simulink model "PhyMod_OpModeSelect"  (R2016b)
settings: configuration reference "CodeGenConfigSet" (kept outside this file)
settings Model: Creator=Administrator  LastModifiedBy=Administrator
settings ConfigSetRef: SourceLocation=Base Workspace

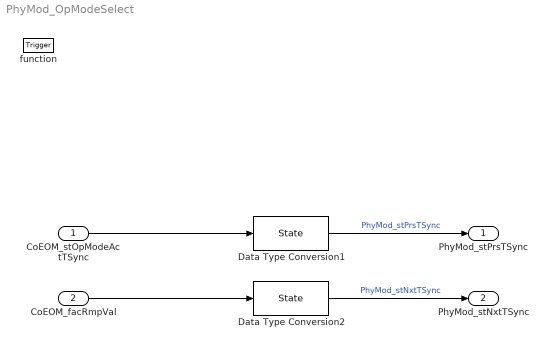
== system PhyMod_OpModeSelect ==
  CoEOM_stOpModeActTSync : Inport  Description=Diesel Particulate Filter Active Regeneration Status  OutMin=0  OutMax=255  OutDataTypeStr=State_uint8
  CoEOM_facRmpVal : Inport  Description=Central ramp value for operation mode change  Port=2  OutMin=-31  OutMax=31  OutDataTypeStr=Factor
  function : TriggerPort  TriggerType=function-call  VariantControl=Variant
  Data Type Conversion1 : DataTypeConversion  OutDataTypeStr=State
  Data Type Conversion2 : DataTypeConversion  OutDataTypeStr=State
  PhyMod_stPrsTSync : Outport  Description=Current operating mode for the torque structure (time synchronous)  OutMin=0  OutMax=255  OutDataTypeStr=State_uint8
  PhyMod_stNxtTSync : Outport  Description=Next operating mode for the torque structure (time synchronous)  Port=2  OutMin=0  OutMax=255  OutDataTypeStr=State_uint8
  wires:
  Data Type Conversion1/1 -> PhyMod_stPrsTSync/1  "PhyMod_stPrsTSync"
  CoEOM_stOpModeActTSync/1 -> Data Type Conversion1/1
  CoEOM_facRmpVal/1 -> Data Type Conversion2/1
  Data Type Conversion2/1 -> PhyMod_stNxtTSync/1  "PhyMod_stNxtTSync"
